simulink model "kalman_verification"  (R2015b)
settings: Solver=ode1  StartTime=0.0  StopTime=30  FixedStep=0.002  RelTol=1e-3
values from neighbouring files (symbols this model uses):
  logts = log.time    [ctr_sim_prepare_ws.m]
  logvals = zeros(numel(logts), n_signals)    [ctr_sim_prepare_ws.m]
libraries: simulink x1
settings Model: Creator=Robert  LastModifiedBy=Robert

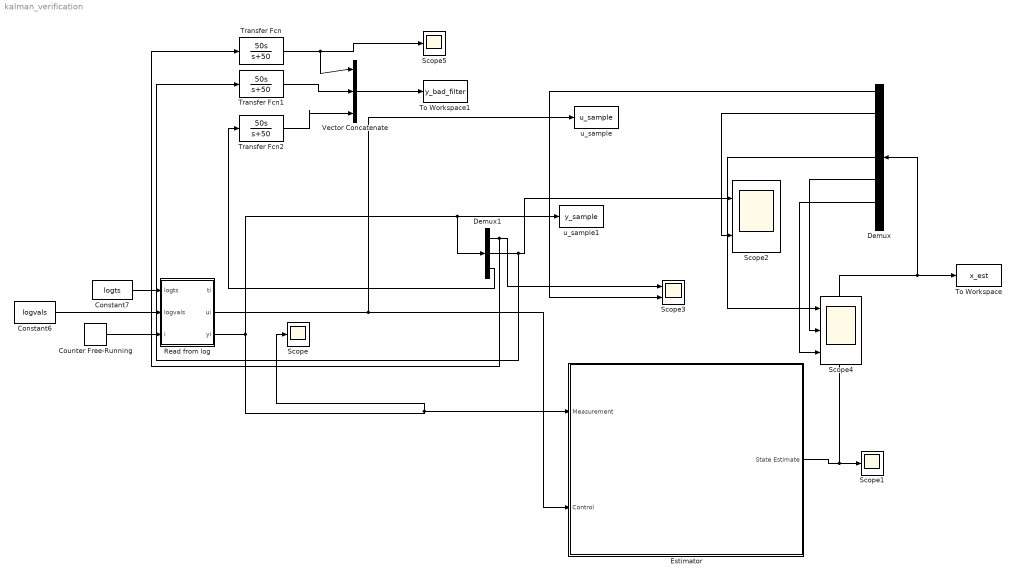
== system kalman_verification ==
  Constant6 : Constant  Value=logvals
  Constant7 : Constant  Value=logts
  Counter Free-Running : simulink/Sources/Counter Free-Running  NumBits=32  tsamp=-1
  Demux : Demux  Outputs=7
  Demux1 : Demux  Outputs=3
  Estimator : Subsystem  mask(Extended Kalman Filter){x0=[ 0.11; 0.11; 0; 0; 0; 0; deg2rad(6) ], P_diag=[1, 1, 1, 1, 1, 1, 1], N_diag=[ 100, 100 ], W_diag=[ 0.0001, 0.00001, 0.00001 ], step_width=0.002}
      mask help: Estimates system state based on measured system inputs, outputs, and knowledge about associated noise parameters.
      mask DialogControl Control2 Prompt: x0:
      mask DialogControl Control3 Prompt: diag(P):
      mask DialogControl Control4 Prompt: diag(N):
      mask DialogControl Control5 Prompt: diag(W):
      mask DialogControl Control6 Prompt: step width:
      mask Display:
      | disp('Extended Kalman Filter')
      | port_label('output', 1, 'State Estimate')
      | port_label('input', 1, 'Measurement')
      | port_label('input', 2, 'Control')
  Read from log : MATLAB Function  TreatAsAtomicUnit=on
  Scope : Scope
  Scope1 : Scope
  Scope2 : Scope  NumInputPorts=2
  Scope3 : Scope  NumInputPorts=2
  Scope4 : Scope  NumInputPorts=3
  Scope5 : Scope
  To Workspace : ToWorkspace  VariableName=x_est  SaveFormat=Structure With Time  SampleTime=-1
  To Workspace1 : ToWorkspace  VariableName=y_bad_filter  SaveFormat=Structure With Time  SampleTime=-1
  Transfer Fcn : TransferFcn  Numerator=[50 0]  Denominator=[1 50]
  Transfer Fcn1 : TransferFcn  Numerator=[50 0]  Denominator=[1 50]
  Transfer Fcn2 : TransferFcn  Numerator=[50 0]  Denominator=[1 50]
  Vector Concatenate : Concatenate  NumInputs=3
  u_sample : ToWorkspace  VariableName=u_sample  SaveFormat=Structure With Time  SampleTime=-1
  u_sample1 : ToWorkspace  VariableName=y_sample  SaveFormat=Structure With Time  SampleTime=-1
  wires:
  Counter Free-Running/1 -> Read from log/3(i)
  Constant6/1 -> Read from log/2(logvals)
  Constant7/1 -> Read from log/1(logts)
  Read from log/3(yi) -> Scope/1, Estimator/1(Measurement), Demux1/1, u_sample1/1
  Read from log/2(ui) -> u_sample/1, Estimator/2(Control)
  Estimator/1(State Estimate) -> Demux/1, To Workspace/1, Scope1/1
  Demux1/2 -> Transfer Fcn1/1, Scope2/1
  Demux/2 -> Scope2/2
  Demux1/1 -> Transfer Fcn/1, Scope3/1
  Demux/1 -> Scope3/2
  Demux/4 -> Scope4/1
  Demux/5 -> Scope4/2
  Demux/6 -> Scope4/3
  Transfer Fcn/1 -> Vector Concatenate/1, Scope5/1
  Demux1/3 -> Transfer Fcn2/1
  Transfer Fcn1/1 -> Vector Concatenate/2
  Transfer Fcn2/1 -> Vector Concatenate/3
  Vector Concatenate/1 -> To Workspace1/1

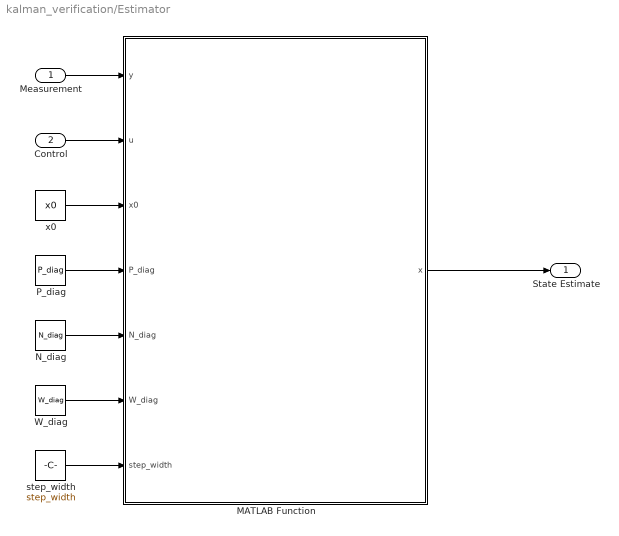
== system kalman_verification/Estimator ==
  Measurement : Inport
  Control : Inport  Port=2
  MATLAB Function : MATLAB Function  TreatAsAtomicUnit=on
  N_diag : Constant  Value=N_diag
  P_diag : Constant  Value=P_diag
  W_diag : Constant  Value=W_diag
  step_width : Constant  Value=step_width
  x0 : Constant  Value=x0
  State Estimate : Outport
  wires:
  MATLAB Function/1(x) -> State Estimate/1
  Measurement/1 -> MATLAB Function/1(y)
  Control/1 -> MATLAB Function/2(u)
  x0/1 -> MATLAB Function/3(x0)
  step_width/1 -> MATLAB Function/7(step_width)
  W_diag/1 -> MATLAB Function/6(W_diag)
  N_diag/1 -> MATLAB Function/5(N_diag)
  P_diag/1 -> MATLAB Function/4(P_diag)

== matlab function kalman_verification/Read from log ==
  data: logts input; logvals input; ti output size=1; ui output; yi output; i input
function [ti, ui, yi] = fcn(logts, logvals, i)
t_start = 12;
i = i + 1 + t_start*500;
ti = logts(i);
ui = logvals(i, 1:2)'; 
yi = logvals(i, 3:5)';

== matlab function kalman_verification/Estimator/MATLAB Function ==
  data: y input; u input; x output; x0 input; P_diag input; N_diag input; W_diag input; step_width input
function x = fcn(y, u, x0, P_diag, N_diag, W_diag, step_width)
persistent sys

if isempty(sys)
    sys = ExtendedKalmanFilter();
    sys.x0 = x0;
    sys.P_diag = P_diag;
    sys.N_diag = N_diag;
    sys.W_diag = W_diag;
    sys.step_width = step_width;
    
    sys.setup(y, u)
    sys.reset()
end

x = sys.step(y, u);
